simulink model "singlephase_half_converterdcmachine"  (R2024b)
settings: Solver=VariableStepAuto  StartTime=0.0  StopTime=0.1  RelTol=1e-3
libraries: spsDiodeLib x2, spsThyristorLib x2, spsVoltageMeasurementLib x2, spsACVoltageSourceLib x1, spsDCMachineLib x1, spsDCVoltageSourceLib x1, sps_lib x1
settings Model: Creator=jangr  LastModifiedBy=harsh

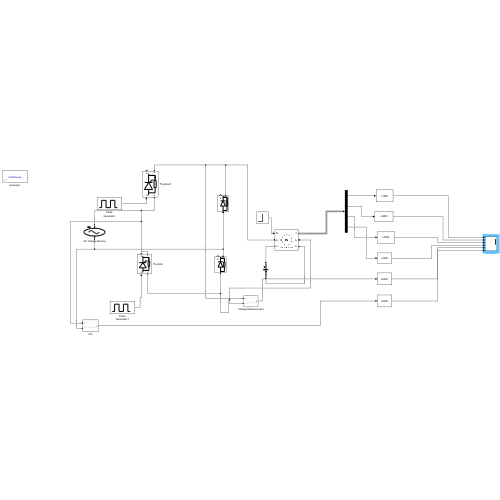
[thumbnail: Simulink's stored preview of the top-level diagram]
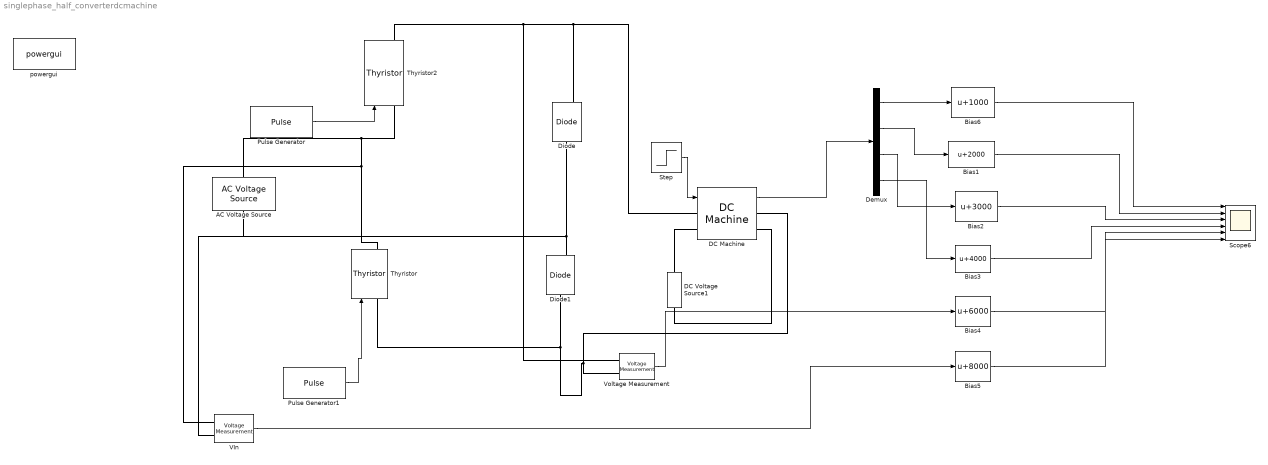
== system singlephase_half_converterdcmachine ==
  AC Voltage Source : spsACVoltageSourceLib/AC Voltage Source  Amplitude=230  Phase=0  Frequency=50  SampleTime=0  Measurements=None  BusType=swing  Pref=10e3  Qref=0  Qmin=-inf  Qmax=+inf
  Bias1 : Bias  Bias=2000  SaturateOnIntegerOverflow=off
  Bias2 : Bias  Bias=3000  SaturateOnIntegerOverflow=off
  Bias3 : Bias  Bias=4000  SaturateOnIntegerOverflow=off
  Bias4 : Bias  Bias=6000  SaturateOnIntegerOverflow=off
  Bias5 : Bias  Bias=8000  SaturateOnIntegerOverflow=off
  Bias6 : Bias  Bias=1000  SaturateOnIntegerOverflow=off
  DC Machine : spsDCMachineLib/DC Machine  PresetModel=No  MechanicalLoad=Torque TL  FieldType=Wound  ShowDetailedParameters=on  MeasurementBus=off  RLa="[ 0.6  0.012]"  RLf="[ 240  120]"  Laf=1.8  MachineConstant=Torque constant (N.m/A)  Ke=1.8  Kt=1.8  J=1  Bm=0  Tf=0  w0=1  Ifinit=0.416666666255433  TsPowergui=0  TsBlock=-1
  DC Voltage Source1 : spsDCVoltageSourceLib/DC Voltage Source  Amplitude=100  Measurements=None
  Demux : Demux
  Diode : spsDiodeLib/Diode  Ron=0.001  Lon=0  Vf=0.8  IC=0  UseSnubber=0  Rs=500  Cs=250e-9  Measurements=on
  Diode1 : spsDiodeLib/Diode  Ron=0.001  Lon=0  Vf=0.8  IC=0  UseSnubber=0  Rs=500  Cs=250e-9  Measurements=on
  Pulse Generator : DiscretePulseGenerator  PulseType=Time based  Period=0.02  PulseWidth=5  PhaseDelay=30*0.02/360
  Pulse Generator1 : DiscretePulseGenerator  PulseType=Time based  Period=0.02  PulseWidth=5  PhaseDelay=210*0.02/360
  Scope6 : Scope  NumInputPorts=6
  Step : Step  SampleTime=0
  Thyristor : spsThyristorLib/Thyristor  Ron=0.001  Lon=0  Vf=0.8  IC=0  Rs=500  Cs=250e-9  Measurements=on
  Thyristor2 : spsThyristorLib/Thyristor  Ron=0.001  Lon=0  Vf=0.8  IC=0  Rs=500  Cs=250e-9  Measurements=on
  VIn : spsVoltageMeasurementLib/Voltage Measurement  PhasorSimulation=off  OutputType=Complex  PSBequivalent=0
  Voltage Measurement : spsVoltageMeasurementLib/Voltage Measurement  PhasorSimulation=off  OutputType=Complex  PSBequivalent=0
  powergui : sps_lib/powergui  Priority=1  SimulationMode=Continuous  SampleTime=50e-6  frequency=60  Iterations=50  frequencyindice=0  Pbase=100e6  ErrMax=1e-4  UnitsV=kV  UnitsW=MW  buscounter=0  FunctionMessages=off  echomessages=off  EnableUseOfTLC=off  CurrentSourceSwitches=off  DisableSnubberDevices=off  DisableRonSwitches=off  DisableVfSwitches=off  DisplayEquations=off  AutomaticDiscreteSolvers=off  SolverType=Tustin/Backward Euler (TBE)  Interpol=off  ExternalGateDelay=off  methode=off  Ts=100  x0status=blocks  SPID=on  SwTol=0  HookPort=off  NonlinearTolerance=1e-4  nMaxIteration=100  ContinueOnMaxIteration=off  RestoreLinks=warning  ResistiveCurrentMeasurement=off  Frange=[0:2:500]  Ylog=off  Xlog=on  ShowGrid=off  save=off  variable=ZData  structure=0  ZoomFFT=off  StartTime=0.0  cycles=1  DisplayStyle=1  fundamental=60  FreqAxis=off  MaxFrequency=1000  frequencyindicesteady=1  RmsSteady=1  display=off
  wires:
  Pulse Generator/1 -> Thyristor2/1
  Pulse Generator1/1 -> Thyristor/1
  Step/1 -> DC Machine/1
  DC Machine/1 -> Demux/1
  Demux/1 -> Bias6/1
  Demux/2 -> Bias1/1
  Demux/3 -> Bias2/1
  Demux/4 -> Bias3/1
  VIn/1 -> Bias5/1
  Voltage Measurement/1 -> Bias4/1
  Bias6/1 -> Scope6/1
  Bias1/1 -> Scope6/2
  Bias2/1 -> Scope6/3
  Bias3/1 -> Scope6/4
  Bias4/1 -> Scope6/5
  Bias5/1 -> Scope6/6
  connections:
  Thyristor2/LConn1 -- AC Voltage Source/RConn1 -- Thyristor/RConn1 -- VIn/LConn1
  VIn/LConn2 -- AC Voltage Source/LConn1 -- Diode1/RConn1 -- Diode/LConn1
  Thyristor2/RConn1 -- Diode/RConn1 -- DC Machine/LConn1 -- Voltage Measurement/LConn1
  Thyristor/LConn1 -- Diode1/LConn1 -- DC Machine/RConn1 -- Voltage Measurement/LConn2
  DC Voltage Source1/RConn1 -- DC Machine/LConn2
  DC Voltage Source1/LConn1 -- DC Machine/RConn2
